simulink model "LATC_Test_Calc5"  (R2021b)
settings: Solver=FixedStepDiscrete  StartTime=4067.8601  StopTime=4107.8798  FixedStep=0.02  RelTol=1e-3
libraries: simulink x8
(part 1 of 2)
settings Model: DataDictionary=LATC.sldd  Creator=GW00216231  LastModifiedBy=GW00216231
settings SolverCC: AlgebraicLoopSolver=TrustRegion
settings OptimizationCC: DefaultParameterBehavior=Inlined  EnhancedBackFolding=on  PassReuseOutputArgsThreshold=0  OptimizeBlockOrder=speed  DifferentSizesBufferReuse=on  OptimizationCustomize=off
settings DebuggingCC: SignalResolutionControl=TryResolveAllWithWarning  ParameterTunabilityLossMsg=error  SFMachineParentedDataDiag=warning  UnderSpecifiedDimensionMsg=warning
settings SFSimCC: MATLABDynamicMemAlloc=off
settings RTWCC: Description=Vector CANape/vSignalyzer Target (Visual C/C++ Project Makefile)  SystemTargetFile=cnp.tlc  TemplateMakefile=cnp_msdll.tmf
settings CodeAppCC: ForceParamTrailComments=on  OperatorAnnotations=on
settings STFCustomTargetCC: TargetLangStandard=C99 (ISO)  MATLABClassNameForMDSCustomization=Simulink.SoftwareTarget.TargetSpecificTriggerConfigurationBase  SystemTargetFile=cnp.tlc

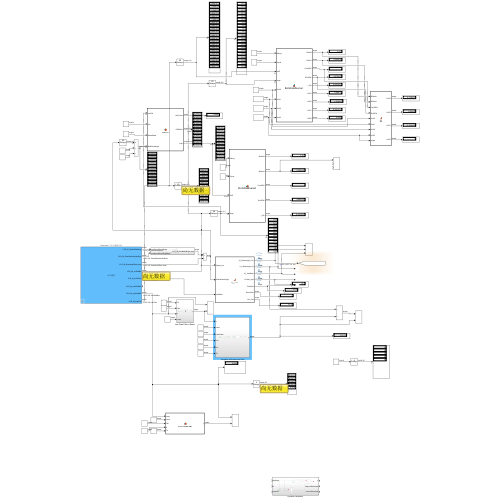
[thumbnail: Simulink's stored preview of the top-level diagram]
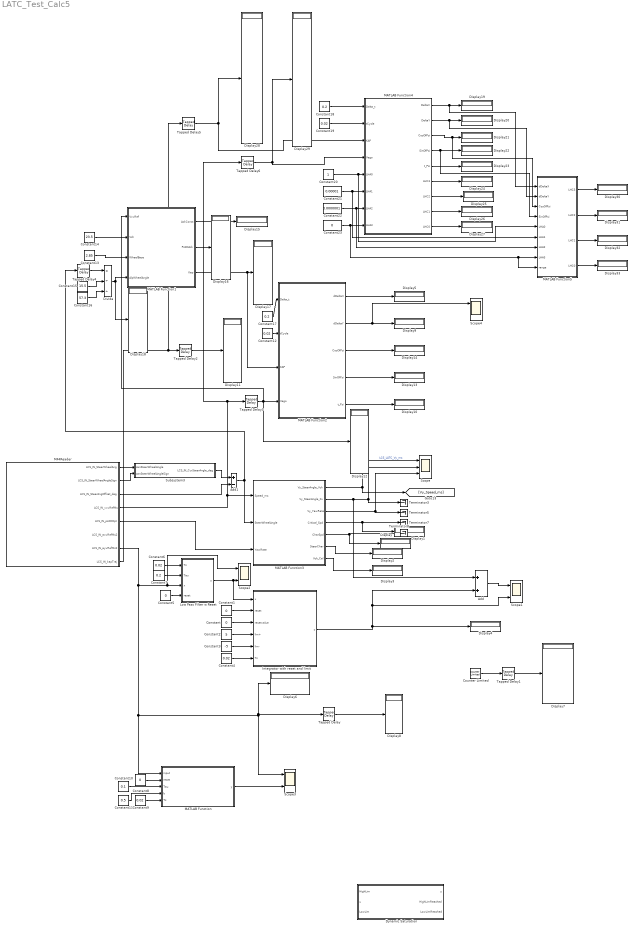
== system LATC_Test_Calc5 ==
  Add : Sum
  Add1 : Sum  Inputs=+-
  Constant{,1,5,8,23} (5 alike) : Constant  Value=0  OutDataTypeStr=single
  Constant10 : Constant  Value=0.1  OutDataTypeStr=single
  Constant11 : Constant  Value=0.5  OutDataTypeStr=single
  Constant{4,6,9,12,19} (5 alike) : Constant  Value=0.02  OutDataTypeStr=single
  Constant13 : Constant  Value=2.85  OutDataTypeStr=single
  Constant14 : Constant  Value=23.5  OutDataTypeStr=single
  Constant15 : Constant  Value=15.5  OutDataTypeStr=single
  Constant16 : Constant  Value=57.3  OutDataTypeStr=single
  Constant17 : Constant  Value=0.2  OutDataTypeStr=single
  Constant18 : Constant  Value=0.2  OutDataTypeStr=single
  Constant2 : Constant  Value=5  OutDataTypeStr=single
  Constant20 : Constant  OutDataTypeStr=single
  Constant21 : Constant  Value=0.00001  OutDataTypeStr=single
  Constant22 : Constant  Value=0.0000001  OutDataTypeStr=single
  Constant3 : Constant  Value=-5  OutDataTypeStr=single
  Constant7 : Constant  Value=0.2  OutDataTypeStr=single
  Counter Limited : simulink/Sources/Counter Limited  uplimit=65535  tsamp=-1
  Display{,1..33} (34 alike) : Display
  Divide : Product  Inputs=*//
  Dynamic Saturation : Subsystem
  Integrator with reset and limit : Subsystem
  Low Pass Filter w Reset : Subsystem
  MATLAB Function : MATLAB Function  TreatAsAtomicUnit=on
  MATLAB Function1 : MATLAB Function  TreatAsAtomicUnit=on
  MATLAB Function2 : MATLAB Function  TreatAsAtomicUnit=on
  MATLAB Function3 : MATLAB Function  TreatAsAtomicUnit=on
  MATLAB Function4 : MATLAB Function  TreatAsAtomicUnit=on
  MATLAB Function5 : MATLAB Function  TreatAsAtomicUnit=on
  MF4Reader : Subsystem  Description=Comment: 汇出有碰撞风险  mask(MF4Reader(Bata1.5)){pfileName=F:\04_APE_Temple_Files\ADAS_CAN+dll+SimulinkModel\TrajectoryPoints_Track_Test4\Data_Recorder\NOH_IDC_V71_0049_2022-05-27-19-39-31.mf4, LoadFilter={'Checksum','RollingCounter','AEB','HAVP_','^P_','BSW','Reserved','PACK','autosar','LM_','exec','fid_stat','g_swc','_PIL_','_TLJ_','_PP_','SPID','DMON','gen_init','JAPedObj','^MAC','CAN_DataFrame','DIAG','CAL'}, CaseSensitive=off, AutoDataTypeConvert=off, FunMod=读入模式, SearchSeed=LCS_*kap, BackGroundColorRead=lightBlue, BackGroundColorPort=white, StopTime=4107.8798, StartTime=4067.8601}
      mask prompts: pfileName "mf4文件:"; LoadFilter "加载过滤:"; CaseSensitive "搜索大小写敏感"; AutoDataTypeConvert "自动数据类型转换"; FunMod "模式选择"; SearchSeed "搜索："; StopTime "数据结束时间"; StartTime "数据开始时间"
      mask help: 该模块可将选择的mdf文件中包含的信号以列表形式读取出来，读入模式下，该模块将用户选择的信号读取成matlab时间序列，并导入simulink用于仿真。接口模式下，该模块将以用户选择的信号名添加CANape仿真用接口，用于dll生成（需要安装CANape simulink addon）。点击"帮助"了解更多。
      settings: AttributesFormatString=%<Description>
      mask Help:
      | Version：Bata1.5  Date: 20211012 Editor: Chengzhenning
      | 当前为测试版，可能存在不稳定或性能问题，建议/Bug反馈请联系Editor，谢谢。
      | 
      | 使用简述：
      | Step1:检查加载过滤。(若如特殊需求无需设置此项)
      | Step2:选取MF4文件
      | Setp3:点击Load/Refresh，加载mf4数据中的信号
      | Step4:选取信号（操作同bus selector，支持搜索）
      | Step5:选择模式及是否自动添加数据类型转换
      | Step6:点击Add添加接口
      | 
      | 数据导入：
      | 选择文件：支持mdf mf4文件，支持中文路径
      | 加载过滤：加载过滤是将符合过滤条件(标准matlab正则表达式)的所有信号跳过，过滤后在“全部信号”中无法找到，可配置多个过滤条件，多个条件以元胞数组的形式输入，例如{'表达式1'，'表达式2'} ，可根据情况自行修改。不建议删除默认的加载过滤条件。
      | 
      | 自定义设置项说明：
      | 读入模式：当配置为导入mdf数据后，该模块会将已选择的信号从mdf文件中读取出来，存入base workspace。并在模型中使用fromworkspace调用。
      | 接口模式：当配置为生成ape接口时，将按照已选择的信号名生成ape仿真用接口模块。
      | 自动数据类型转换：设置为自动数据类型转换之后将在内部自动添加data type conversion，请务必规定后端使用的数据类型，否者以读出或输入的数据类型直出。
      | 
      | 搜索：
      | 搜索：搜索支持常用通配符（同ape），当搜索条件为空或点击输入框的取消后将重置搜索结果，搜索条件请在弹出的输入框中输入；
      | 
      | 其他提醒：
      | 因版本限制，自定义设置部分请用右侧按钮进行设置，左侧仅作显示用；
      | 因版本限制，搜索条件请在弹出的输入框中输入；
      | 加载数据后，该模块会自动将仿真起止时间设置为所有有效数据的最大起止时间区间，仿真步长需要自行设置；
      | 
      | 故障解决：
      | 若发生接口混乱的情况，点击不常用设置->ClearPorts！删除所有模块后重新添加。
      | 若存在其他报错问题，尝试执行clear all（所有工作区将被清除，注意保存数据！！！）后重新load数据。
      | 若提醒找不到变，在没有clear all的前提下，重新Add即可。若执行了clear all，需要点击Load重新加载数据。
      | 
      | 兼容性：
      | 兼容20b和21a，但因2020b兼容性问题，部分参数只能使用对话框的形式输入而不能直接修改，Matlab 21a版本体验更佳。若需要21a版，请联系Editor。
      | 
      | 警告：
      | 删除默认的加载过滤条件可能会导致错误，不建议删除默认的加载过滤条件！
      | 每个模型中只能同时使用一个MF4Reader !
      | 尽量不要手动清空工作区，clear之后需求重新add，clear all之后需要重新load并add
      | 
      | 更新记录：
      | 1 Bata1.0  Date 20210927 Editor Chengzhenning
      |    初版发布
      | 2 Bata1.1  Date 20210929 Editor Chengzhenning
      |    优化个别无法读取的信号的检测过滤,提高对数据的兼容性，bug反馈人：温俊亮
      | 3 Bata1.2  Date 20210930 Editor Chengzhenning
      |    修复重调整接口会导致外部连线混乱的问题，不再使用弹窗提醒找不到的信号，bug反馈人：王亚伟
      | 4.Bata1.3  Date 20210930 Editor Chengzhenning
      |    自动添加信号名，提升加载数据速度
      | 5.Bata1.4  Date 20211009 Editor Chengzhenning
      |    增加内部的自动信号类型转换，可配置。支持设置搜索是否大小写敏感。更改设置工作模式的位置，不必每次都设置。
      | 6.Bata1.5  Date 20211012 Editor Chengzhenning
      |    适配2021b，不再兼容2020b以下。其他操作逻辑优化，更易使用。
      | 
      | 感谢所有提供bug反馈和功能建议的用户！
      mask TypeOptions FunMod: 读入模式 | 接口模式
      mask DialogControl ParameterGroupVar Prompt: 数据源选择
      mask DialogControl Control2 Prompt: 选择文件
      mask DialogControl Control2 Callback:
      | global fileobj;
      | 
      | [Name,directory] = uigetfile('*.mf4;*.mdf','Choose a mf4-file');
      | if isequal(Name,0) || isequal(directory,0)
      |     disp('User pressed cancel')
      |     return;
      | else
      |     fName=fullfile(directory,Name);
      |     if strcmp(fName,get_param(gcb,'pfileName'))&&~isempty(fileobj)
      |         return;
      |     end
      |     set_param(gcb,'pfileName',fName);
      |     disp(['User selected ',fName ])
      | end
      | 
      | 
      | commentStr=NaN;
      | StartTime=0;
      | StopTime=30;
      | if ~isempty(Simulink.Mask.get(gcb).Parameters(2).Value)
      |     LoadExclude=eval(Simulink.Mask.get(gcb).Parameters(2).Value);
      |     if ~iscell(LoadExclude)
      |         msgbox('加载过滤必须是元胞字符串数组或空值！');
      |         return;
      |     end
      | else
      |     LoadExclude={};
      | end
      | fName=Simulink.Mask.get(gcb).Parameters(1).Value;
      | if ~exist(fName)
      |     msgbox('文件不存在！');
      |     return;
      | end
      | t1=clock;
      | disp('-----------------------------');
      | disp(['打开文件:',fName,'中...']);
      | bar = waitbar(0,'正在读取数据...0%');
      | fileobj=mdf(fName);
      | disp(['打开完成，用时',num2str(etime(clock,t1)),'秒']);
      | %commentStr=native2unicode(unicode2native(fileobj.Comment,'windows-1252'));%20b以下版本用
      | commentStr=fileobj.Comment;
      | disp(['数据备注:',commentStr]);
      | t1=clock;
      | disp('读取信号中...');
      | ALLSigNames={};
      | ALLSigsGroup={};
      | ChannelNamesNum=length(fileobj.ChannelNames);
      | timeflag=true;
      | for i=2:ChannelNamesNum
      |     if ishandle(bar)
      |         str=['正在加载数据...',num2str(fix(100*i/ChannelNamesNum)),'%'];
      |         waitbar(i/ChannelNamesNum,bar,str,'Interpreter','none');
      |     end
      |     if fileobj.ChannelGroup(i).DataSize==0
      |         continue;
      |     end
      |     for m=1:length(fileobj.ChannelNames{i})
      |         ChannelName=fileobj.ChannelNames{i}{m};
      |         if (ChannelName=='t')
      |             continue;
      |         end
      |         if isempty(ChannelName)
      |             continue;
      |         end
      |         ExcludeFlag=false;
      |         for x=1:length(LoadExclude)
      |             if regexp(ChannelName,LoadExclude{x})
      |                 ExcludeFlag=true;
      |             end
      |         end
      |         if ExcludeFlag
      |             continue;
      |         end
      |         try
      |             temp=read(fileobj,i,ChannelName,'OutputFormat','Timeseries');
      |         catch
      |             disp([ChannelName,'不支持读入,已跳过！']);
      |         end
      |         if isempty(temp)
      |             continue;
      |         end
      |         timelength=temp.TimeInfo.end-temp.TimeInfo.start;
      |         if timelength<=0
      |             continue;
      |         end
      |         if timeflag
      |             StartTime=temp.TimeInfo.start;
      |             StopTime=temp.TimeInfo.end;
      |             timeflag=false;
      |         else
      |             if StartTime>temp.TimeInfo.start
      |                 StartTime=temp.TimeInfo.start;
      |             end
      |             if StopTime<temp.TimeInfo.end
      |                 StopTime=temp.TimeInfo.end;
      |             end
      |         end
      | 
      |         ALLSigNames=[ALLSigNames,ChannelName];
      |         ALLSigsGroup=[ALLSigsGroup,num2str(i)];
      |     end
      | end
      | 
      | %set_param(gcs,'StartTime',num2str(StartTime));
      | %set_param(gcs,'StopTime',num2str(StopTime));
      | set_param(gcb,'StartTime',num2str(StartTime));
      | set_param(gcb,'StopTime',num2str(StopTime));
      | waitbar(1,bar,['加载结束，信号数量：',num2str(length(ALLSigNames))],'Interpreter','none');
      | pause(2);
      | if ishandle(bar)
      |     close(bar);
      | end
      | if isempty(ALLSigNames)
      |     msgbox('读取数据失败！');
      |     disp('异常结束!');
      |     return;
      | else
      |     %commentStr=native2unicode(unicode2native(fileobj.Comment,'windows-1252'));
      |     disp(['读取完成,','信号数量：',num2str(length(ALLSigNames)),',用时',num2str(etime(clock,t1)),'秒']);
      |     disp(['数据起止时间为[',num2str(StartTime),' , ',num2str(StopTime),']']);
      |     disp('Finish!');
      | end
      | disp('-----------------------------');
      | set_param(gcb,'Description',['Comment: ',commentStr]);
      | 
      | 
      | maskObj = Simulink.Mask.get( gcb );
      | ControlALLSigsGroup= maskObj.getDialogControl('ALLSigsGroup');
      | ControlALLSigNames= maskObj.getDialogControl('ALLSigNames');
      | treeControlL = maskObj.getDialogControl('Control3');
      | treeControlR = maskObj.getDialogControl('Control6');
      | 
      | ControlALLSigsGroup.TreeItems=ALLSigsGroup;
      | ControlALLSigNames.TreeItems=ALLSigNames;
      | treeControlL.TreeItems=ALLSigNames;
      | 
      | selAllSig=treeControlR.TreeItems();
      | if isempty(selAllSig)
      |     return;
      | end
      | for i= 1:length(selAllSig)
      |     if max(strfind(selAllSig{i},'???'))>0
      |         if ismember(selAllSig{i}(4:end),ALLSigNames)
      |             selAllSig{i}=selAllSig{i}(4:end);
      |         end
      |     else
      |         if ~ismember(selAllSig{i},ALLSigNames)
      |             selAllSig{i}=['???',selAllSig{i}];
      |         end
      |     end
      | end
      | treeControlR.TreeItems=selAllSig;
      mask DialogControl Container11 Prompt: 自定义设置
      mask DialogControl SearchButton Prompt: Search
      mask DialogControl SearchButton Callback:
      | maskObj = Simulink.Mask.get( gcb );
      | treeControlL = maskObj.getDialogControl('Control3');
      | ControlALLSigNames= maskObj.getDialogControl('ALLSigNames');
      | ALLSigNames=ControlALLSigNames.TreeItems();
      | 
      | SearchSeed= get_param(gcb,'SearchSeed');
      | SearchSeed=strrep(SearchSeed,'[','');
      | SearchSeed=strrep(SearchSeed,']','');
      | SLsiglist={};
      | if isempty(SearchSeed)
      |     treeControlL.TreeItems=ALLSigNames;
      |     return;
      | end
      | CaseSensitive=get_param(gcb,'CaseSensitive');
      | if CaseSensitive=="off"
      |     for i=1:length(ALLSigNames)
      |         if regexpi(ALLSigNames{i},regexptranslate('wildcard',SearchSeed))
      |             %if regexp(ALLSigNames{i},SerchSeed)
      |             SLsiglist=[SLsiglist,ALLSigNames{i}];
      |         end
      |     end
      | else
      |     for i=1:length(ALLSigNames)
      |         if regexp(ALLSigNames{i},regexptranslate('wildcard',SearchSeed))
      |         %   if regexp(ALLSigNames{i},SerchSeed)
      |             SLsiglist=[SLsiglist,ALLSigNames{i}];
      |         end
      |     end
      | end
      | treeControlL.TreeItems=SLsiglist;
      mask DialogControl Control3 Prompt: 所有信号
      mask DialogControl Control9 Prompt: Load
      mask DialogControl Control9 Callback:
      | global fileobj;
      | 
      | commentStr=NaN;
      | StartTime=0;
      | StopTime=30;
      | if ~isempty(Simulink.Mask.get(gcb).Parameters(2).Value)
      |     LoadExclude=eval(Simulink.Mask.get(gcb).Parameters(2).Value);
      |     if ~iscell(LoadExclude)
      |         msgbox('加载过滤必须是元胞字符串数组或空值！');
      |         return;
      |     end
      | else
      |     LoadExclude={};
      | end
      | fName=Simulink.Mask.get(gcb).Parameters(1).Value;
      | if ~exist(fName)
      |     msgbox('文件不存在！');
      |     return;
      | end
      | t1=clock;
      | disp('-----------------------------');
      | disp(['打开文件:',fName,'中...']);
      | bar = waitbar(0,'正在读取数据...0%');
      | fileobj=mdf(fName);
      | disp(['打开完成，用时',num2str(etime(clock,t1)),'秒']);
      | %commentStr=native2unicode(unicode2native(fileobj.Comment,'windows-1252'));%20b以下版本用
      | commentStr=fileobj.Comment;
      | disp(['数据备注:',commentStr]);
      | t1=clock;
      | disp('读取信号中...');
      | ALLSigNames={};
      | ALLSigsGroup={};
      | ChannelNamesNum=length(fileobj.ChannelNames);
      | timeflag=true;
      | for i=2:ChannelNamesNum
      |     if ishandle(bar)
      |         str=['正在加载数据...',num2str(fix(100*i/ChannelNamesNum)),'%'];
      |         waitbar(i/ChannelNamesNum,bar,str,'Interpreter','none');
      |     end
      |     if fileobj.ChannelGroup(i).DataSize==0
      |         continue;
      |     end
      |     for m=1:length(fileobj.ChannelNames{i})
      |         ChannelName=fileobj.ChannelNames{i}{m};
      |         if (ChannelName=='t')
      |             continue;
      |         end
      |         if isempty(ChannelName)
      |             continue;
      |         end
      |         ExcludeFlag=false;
      |         for x=1:length(LoadExclude)
      |             if regexp(ChannelName,LoadExclude{x})
      |                 ExcludeFlag=true;
      |             end
      |         end
      |         if ExcludeFlag
      |             continue;
      |         end
      |         try
      |             temp=read(fileobj,i,ChannelName,'OutputFormat','Timeseries');
      |         catch
      |             disp([ChannelName,'不支持读入,已跳过！']);
      |         end
      |         if isempty(temp)
      |             continue;
      |         end
      |         timelength=temp.TimeInfo.end-temp.TimeInfo.start;
      |         if timelength<=0
      |             continue;
      |         end
      |         if timeflag
      |             StartTime=temp.TimeInfo.start;
      |             StopTime=temp.TimeInfo.end;
      |             timeflag=false;
      |         else
      |             if StartTime>temp.TimeInfo.start
      |                 StartTime=temp.TimeInfo.start;
      |             end
      |             if StopTime<temp.TimeInfo.end
      |                 StopTime=temp.TimeInfo.end;
      |             end
      |         end
      | 
      |         ALLSigNames=[ALLSigNames,ChannelName];
      |         ALLSigsGroup=[ALLSigsGroup,num2str(i)];
      |     end
      | end
      | 
      | %set_param(gcs,'StartTime',num2str(StartTime));
      | %set_param(gcs,'StopTime',num2str(StopTime));
      | set_param(gcb,'StartTime',num2str(StartTime));
      | set_param(gcb,'StopTime',num2str(StopTime));
      | waitbar(1,bar,['加载结束，信号数量：',num2str(length(ALLSigNames))],'Interpreter','none');
      | pause(2);
      | if ishandle(bar)
      |     close(bar);
      | end
      | if isempty(ALLSigNames)
      |     msgbox('读取数据失败！');
      |     disp('异常结束!');
      |     return;
      | else
      |     %commentStr=native2unicode(unicode2native(fileobj.Comment,'windows-1252'));
      |     disp(['读取完成,','信号数量：',num2str(length(ALLSigNames)),',用时',num2str(etime(clock,t1)),'秒']);
      |     disp(['数据起止时间为[',num2str(StartTime),' , ',num2str(StopTime),']']);
      |     disp('Finish!');
      | end
      | disp('-----------------------------');
      | set_param(gcb,'Description',['Comment: ',commentStr]);
      | 
      | 
      | maskObj = Simulink.Mask.get( gcb );
      | ControlALLSigsGroup= maskObj.getDialogControl('ALLSigsGroup');
      | ControlALLSigNames= maskObj.getDialogControl('ALLSigNames');
      | treeControlL = maskObj.getDialogControl('Control3');
      | treeControlR = maskObj.getDialogControl('Control6');
      | 
      | ControlALLSigsGroup.TreeItems=ALLSigsGroup;
      | ControlALLSigNames.TreeItems=ALLSigNames;
      | treeControlL.TreeItems=ALLSigNames;
      | 
      | selAllSig=treeControlR.TreeItems();
      | if isempty(selAllSig)
      |     return;
      | end
      | for i= 1:length(selAllSig)
      |     if max(strfind(selAllSig{i},'???'))>0
      |         if ismember(selAllSig{i}(4:end),ALLSigNames)
      |             selAllSig{i}=selAllSig{i}(4:end);
      |         end
      |     else
      |         if ~ismember(selAllSig{i},ALLSigNames)
      |             selAllSig{i}=['???',selAllSig{i}];
      |         end
      |     end
      | end
      | treeControlR.TreeItems=selAllSig;
      mask DialogControl Control7 Prompt: Select >>
      mask DialogControl Control7 Callback:
      | maskObj = Simulink.Mask.get( gcb );
      | treeControlL = maskObj.getDialogControl('Control3');
      | treeControlR = maskObj.getDialogControl('Control6');
      | 
      | seld=treeControlL.getSelectedItems();
      | if isempty(seld)
      |     return;
      | end
      | if ismember(seld,treeControlR.TreeItems)
      |     msgbox('信号重复')
      | end
      | treeControlR.TreeItems=unique([treeControlR.TreeItems,seld'],'stable');
      | treeControlR.setSelectedItems(seld);
      mask DialogControl Control6 Prompt: 已选信号
      mask DialogControl up Prompt: Up
      mask DialogControl up Callback:
      | maskObj = Simulink.Mask.get(gcb);
      | treeControlR = maskObj.getDialogControl('Control6');
      | RSig=treeControlR.TreeItems();
      | SelectSig=treeControlR.getSelectedItems();
      | 
      | if isempty(SelectSig)
      |     return;
      | end
      | 
      | [~,selIndex]=ismember(SelectSig,RSig);
      | 
      | if min(selIndex)>2
      |     AllSigPart3=RSig(1:min(selIndex)-2);
      | else
      |     AllSigPart3={};
      | end
      | RSig(selIndex)=[];
      | [~,Part1Index]=ismember(AllSigPart3,RSig);
      | RSig(Part1Index)=[];
      | 
      | treeControlR.TreeItems=[AllSigPart3,SelectSig',RSig];
      | treeControlR.setSelectedItems(SelectSig);
      mask DialogControl down Prompt: Down
      mask DialogControl down Callback:
      | maskObj = Simulink.Mask.get(gcb);
      | treeControlR = maskObj.getDialogControl('Control6');
      | RSig=treeControlR.TreeItems();
      | SelectSig=treeControlR.getSelectedItems();
      | 
      | if isempty(SelectSig)
      |     return;
      | end
      | 
      | [~,selIndex]=ismember(SelectSig,RSig);
      | 
      | if max(selIndex)+2<=length(RSig)
      |     AllSigPart3=RSig(max(selIndex)+2:end);
      | else
      |     AllSigPart3={};
      | end
      | RSig(selIndex)=[];
      | [~,Part3Index]=ismember(AllSigPart3,RSig);
      | RSig(Part3Index)=[];
      | 
      | treeControlR.TreeItems=[RSig,SelectSig',AllSigPart3];
      | treeControlR.setSelectedItems(SelectSig);
      mask DialogControl Control11 Prompt: Remove
      mask DialogControl Control11 Callback:
      | maskObj = Simulink.Mask.get(gcb);
      | treeControlR = maskObj.getDialogControl('Control6');
      | AllSig=treeControlR.TreeItems();
      | SelectSig=treeControlR.getSelectedItems();
      | if ~isempty(SelectSig)
      |     [~,DelIndex]=ismember(SelectSig,AllSig);
      |     AllSig(DelIndex)=[];
      | end
      | treeControlR.TreeItems=AllSig;
      mask DialogControl Control8 Prompt: Add
      mask DialogControl Control8 Callback:
      | global fileobj
      | if isempty(fileobj)
      |     msgbox('数据丢失，请重新load！');
      |     return;
      | end
      | FunMod=get_param(gcb,'FunMod');
      | %检查是否存在未识别到的信号
      | maskObj = Simulink.Mask.get( gcb );
      | treeControlL = maskObj.getDialogControl('Control3');
      | treeControlR = maskObj.getDialogControl('Control6');
      | ControlALLSigsGroup= maskObj.getDialogControl('ALLSigsGroup');
      | ControlALLSigNames= maskObj.getDialogControl('ALLSigNames');
      | ControlOldSigName= maskObj.getDialogControl('OldSigName');
      | 
      | DataSelect=treeControlR.TreeItems();
      | ALLSigsGroup=ControlALLSigsGroup.TreeItems();
      | ALLSigNames=ControlALLSigNames.TreeItems();
      | OldSigName=ControlOldSigName.TreeItems();
      | 
      | if isempty(DataSelect)
      |     msgbox('未选择信号！');
      |     return;
      | end
      | if isempty(DataSelect)
      |     return;
      | end
      | if ~iscell(ALLSigNames)
      |     ALLSigNames={};
      | end
      | for i= 1:length(DataSelect)
      |     if max(strfind(DataSelect{i},'???'))>0
      |         if ismember(DataSelect{i}(4:end),ALLSigNames)
      |             DataSelect{i}=DataSelect{i}(4:end);
      |         end
      |     else
      |         if ~ismember(DataSelect{i},ALLSigNames)
      |             DataSelect{i}=['???',DataSelect{i}];
      |         end
      |     end
      | end
      | treeControlR.TreeItems=DataSelect;
      | signotfind=false;
      | for i= 1:length(DataSelect)
      |     if max(strfind(DataSelect{i},'???'))>0
      |         signotfind=true;
      |     end
      | end
      | if signotfind
      |     signotfindresp=questdlg('存在已选的信号无法找到！请刷新数据或检查数据中是否存在这些信号','错误提醒','跳过无法找到的信号','停止添加接口','停止添加接口');
      |     if isempty(signotfindresp) || signotfindresp == "停止添加接口"
      |         return;
      |     end
      | end
      | 
      | oldPos=get_param(gcb,'Position');%记忆位置，防止游走
      | %定义模块路径方便使用
      | FunctionBlockPath = 'simulink/User-Defined Functions/Interpreted MATLAB Function';
      | OutPortBlockPath ='simulink/Commonly Used Blocks/Out1';
      | SaturationPath ='simulink/Discontinuities/Saturation';
      | ConstantPath = 'simulink/Sources/Constant';
      | DIPath = 'simulink/Discrete/Discrete-Time Integrator';
      | FromWorkSpacePath = 'simulink/Sources/From Workspace';
      | CANapeInputPath='canapelib/CANape I//O/Input';
      | DataTypeConversionPath='simulink/Signal Attributes/Data Type Conversion';
      | 
      | %添加模块前先删除所有模块和连线
      | set_param(gcb,'BackGroundColor','white');
      | SourceList=find_system(gcb,'LookUnderMasks','on','SearchDepth',1,'BlockType','FromWorkspace');
      | if ~isempty(SourceList)
      |     for i=1:length(SourceList)
      |         delete_block(SourceList{i});
      |     end
      | end
      | LinesList=find_system(gcb,'LookUnderMasks','on','FindAll','on','type','line');
      | if ~isempty(LinesList)
      |     for i=1:length(LinesList)
      |         if ishandle(LinesList(i))
      |             delete_line(LinesList(i));
      |         end
      |     end
      | end
      | 
      | SysList=find_system(gcb,'LookUnderMasks','on','SearchDepth',1,'BlockType','SubSystem');
      | if length(SysList)>1
      |     for i=2:length(SysList)
      |         delete_block(SysList{i});
      |     end
      | end
      | DataTypeConversionsList=find_system(gcb,'LookUnderMasks','on','SearchDepth',1,'BlockType','DataTypeConversion');
      | if ~isempty(DataTypeConversionsList)
      |     for i=1:length(DataTypeConversionsList)
      |         delete_block(DataTypeConversionsList{i});
      |     end
      | end
      | %添加信号源
      | SourceBlockSum=0;
      | added_block={};
      | if ~isempty(OldSigName)
      |     for i=1:length(OldSigName);
      |         evalin('base',['clear ',OldSigName{i}]);
      |     end
      | end
      | AutoDataTypeConvert=get_param(gcb,'AutoDataTypeConvert');
      | 
      | if FunMod=="读入模式" %fromworkspace
      |     for j=1:length(DataSelect)
      |         SigName=DataSelect{j};
      |         temp=strrep(SigName,'.','_');
      |         temp=strrep(temp,'[','_');
      |         temp=strrep(temp,']','_');
      |         if length(temp)>60
      |             temp=temp(length(temp)-59:end);
      |         end
      |         SigAliasName=['s_',temp];
      |         [SigExist,Sigindex]= ismember(SigName,ALLSigNames);
      |         if SigExist
      |             sigGroupIndex=str2double(ALLSigsGroup{Sigindex});
      |         else
      |             disp(['未找到信号: ',SigName,' ，已跳过！']);
      |             continue;
      |         end
      |         %添加模块
      |         Swidth=100;
      |         Shigh=30;
      |         Owidth=30;
      |         Ohigh=14;
      |         Sdy=30;
      |         SOdx=800;
      |         SDdx=250;
      |         temp=read(fileobj,sigGroupIndex,SigName,'OutputFormat','Timeseries');
      |         assignin('base',SigAliasName,temp);
      |         Source=add_block(FromWorkSpacePath,[gcb,'/' ,'sourceValue_',SigName],'Interpolate','off','VariableName',SigAliasName,'OutputAfterFinalValue','Setting to zero', ...
      |             'Position',[0,(Shigh)*SourceBlockSum+SourceBlockSum*Sdy, Swidth ,(Shigh)*(SourceBlockSum+1)+SourceBlockSum*Sdy]);
      |         if AutoDataTypeConvert=="on"
      |             DataTypeConversion=add_block(DataTypeConversionPath,[gcb,'/' ,'Convert_',SigName], ...
      |                 'Position',[SDdx,(Shigh)*SourceBlockSum+SourceBlockSum*Sdy, SDdx+Swidth ,(Shigh)*(SourceBlockSum+1)+SourceBlockSum*Sdy]);
      |         end
      |         Out=find_system(gcb,'LookUnderMasks','on','SearchDepth',1,'BlockType','Outport','PortName',SigName);
      |         if isempty(Out)
      |             Out=add_block(OutPortBlockPath,[gcb,'/' ,SigName],...
      |                 'Position',[SOdx,0.5*(Shigh-Ohigh)+(Ohigh)*SourceBlockSum+SourceBlockSum*(Sdy+Shigh-Ohigh),SOdx+Owidth ,0.5*(Shigh-Ohigh)+(Ohigh)*(SourceBlockSum+1)+SourceBlockSum*(Sdy+Shigh-Ohigh)]);
      |         else
      |             Out=Out{1};
      |             set_param(Out,'Port',num2str(SourceBlockSum+1),'Position',[SOdx,0.5*(Shigh-Ohigh)+(Ohigh)*SourceBlockSum+SourceBlockSum*(Sdy+Shigh-Ohigh),SOdx+Owidth ,0.5*(Shigh-Ohigh)+(Ohigh)*(SourceBlockSum+1)+SourceBlockSum*(Sdy+Shigh-Ohigh)]);
      |         end
      |         if AutoDataTypeConvert=="on"
      |             add_line(gcb,get_param(Source,'PortHandles').Outport,get_param(DataTypeConversion,'PortHandles').Inport)
      |             line=add_line(gcb,get_param(DataTypeConversion,'PortHandles').Outport,get_param(Out,'PortHandles').Inport);
      |         else
      |             line=add_line(gcb,get_param(Source,'PortHandles').Outport,get_param(Out,'PortHandles').Inport);
      |         end
      |         set_param(line,'Name',SigName);
      |         SourceBlockSum=SourceBlockSum+1;
      |         set_param(get_param(gcb,'PortHandles').Outport(SourceBlockSum),'ShowPropagatedSignals','on');
      |         OldSigName{j}=SigAliasName;
      |     end
      |     set_param(gcb,'BackGroundColor',get_param(gcb,'BackGroundColorRead'));
      |     set_param(gcs,'StartTime',get_param(gcb,'StartTime'));
      |     set_param(gcs,'StopTime',get_param(gcb,'StopTime'));
      |     disp('读入数据完成，已经自动设置模型仿真时间为数据起止时间');
      | elseif FunMod=="接口模式"
      |     for j=1:length(DataSelect)
      |         SigName=DataSelect{j};
      |         temp=strrep(SigName,'.','_');
      |         if length(temp)>60
      |             temp=temp(length(temp)-59:end);
      |         end
      |         SigAliasName=['s_',temp];
      |         [SigExist,Sigindex]= ismember(SigName,ALLSigNames);
      |         if SigExist
      |             sigGroupIndex=ALLSigsGroup{Sigindex};
      |         else
      |             disp(['未找到信号: ',SigName,' ，已跳过！']);
      |             continue
      |         end
      |         %添加模块
      |         Swidth=100;
      |         Shigh=30;
      |         Owidth=30;
      |         Ohigh=14;
      |         Sdy=30;
      |         SOdx=800;
      |         SDdx=250;
      |         try
      |         Source=add_block('canapelib/CANape I//O/Input',[gcb,'/' ,'sourceValue_',SigName],...
      |             'envName',SigName,'Position',[0,(Shigh)*SourceBlockSum+SourceBlockSum*Sdy, Swidth ,(Shigh)*(SourceBlockSum+1)+SourceBlockSum*Sdy]);
      |         catch
      |             msgbox('可能未安装CANape Simulink Add-on！无法添加接口，已终止！')
      |             return;
      |         end
      |         if AutoDataTypeConvert=="on"
      |             DataTypeConversion=add_block(DataTypeConversionPath,[gcb,'/' ,'Convert_',SigName], ...
      |                 'Position',[SDdx,(Shigh)*SourceBlockSum+SourceBlockSum*Sdy-10, SDdx+Swidth ,(Shigh)*(SourceBlockSum+1)+SourceBlockSum*Sdy-10]);
      |         end
      |         Out=find_system(gcb,'LookUnderMasks','on','SearchDepth',1,'BlockType','Outport','PortName',SigName);
      |         if isempty(Out)
      |             Out=add_block(OutPortBlockPath,[gcb,'/' ,SigName],...
      |                 'Position',[SOdx,0.5*(Shigh-Ohigh)+(Ohigh)*SourceBlockSum+SourceBlockSum*(Sdy+Shigh-Ohigh)-10,SOdx+Owidth ,0.5*(Shigh-Ohigh)+(Ohigh)*(SourceBlockSum+1)+SourceBlockSum*(Sdy+Shigh-Ohigh)-10]);
      |         else
      |             Out=Out{1};
      |             set_param(Out,'Port',num2str(SourceBlockSum+1),'Position',[SOdx,0.5*(Shigh-Ohigh)+(Ohigh)*SourceBlockSum+SourceBlockSum*(Sdy+Shigh-Ohigh)-10,SOdx+Owidth ,0.5*(Shigh-Ohigh)+(Ohigh)*(SourceBlockSum+1)+SourceBlockSum*(Sdy+Shigh-Ohigh)-10]);
      |         end
      |         if AutoDataTypeConvert=="on"
      |             add_line(gcb,get_param(Source,'PortHandles').Outport(1),get_param(DataTypeConversion,'PortHandles').Inport)
      |             line=add_line(gcb,get_param(DataTypeConversion,'PortHandles').Outport,get_param(Out,'PortHandles').Inport);
      |         else
      |             line=add_line(gcb,get_param(Source,'PortHandles').Outport(1),get_param(Out,'PortHandles').Inport);
      |         end
      |         set_param(line,'Name',SigName);
      |         SourceBlockSum=SourceBlockSum+1;
      |         set_param(get_param(gcb,'PortHandles').Outport(SourceBlockSum),'ShowPropagatedSignals','on');
      |         OldSigName{j}=SigAliasName;
      |     end
      |     set_param(gcb,'BackGroundColor',get_param(gcb,'BackGroundColorPort'));
      |     set_param(gcs,'StartTime','0');
      |     disp('添加CANape接口完成，已经自动设置模型仿真开始时间为0');
      | end
      | ControlOldSigName.TreeItems=OldSigName;
      | % 删除多余output
      | OutList=find_system(gcb,'LookUnderMasks','on','SearchDepth',1,'BlockType','Outport');
      | if ~isempty(OutList)
      |     for i=1:length(OutList)
      |         if str2double(get_param(OutList{i},'Port'))>SourceBlockSum
      |             delete_block(OutList{i});
      |         end
      |     end
      | end
      | 
      | if (oldPos(4)-oldPos(2))/SourceBlockSum<20
      |     oldPos(4)=oldPos(2)+(SourceBlockSum+1)*20;
      | end
      | set_param(gcb,'Position',oldPos);
      mask DialogControl ccc Prompt: 其他不常用设置
      mask DialogControl Control17 Prompt: 记忆当前模式模块颜色
      mask DialogControl Control17 Callback:
      | FunMod=get_param(gcb,'FunMod');
      | if FunMod=="读入模式"
      |     set_param(gcb,'BackGroundColorRead',get_param(gcb,'BackGroundColor'));
      | end
      | if FunMod=="接口模式"
      |     set_param(gcb,'BackGroundColorPort',get_param(gcb,'BackGroundColor'));
      | end
      mask DialogControl Control25 Prompt: ClearPorts!
      mask DialogControl Control25 Callback:
      | SourceList=find_system(gcb,'LookUnderMasks','on','SearchDepth',1,'BlockType','FromWorkspace');
      | if ~isempty(SourceList)
      |     for i=1:length(SourceList)
      |         delete_block(SourceList{i});
      |     end
      | end
      | LinesList=find_system(gcb,'LookUnderMasks','on','FindAll','on','type','line');
      | if ~isempty(LinesList)
      |     for i=1:length(LinesList)
      |         if ishandle(LinesList(i))
      |             delete_line(LinesList(i));
      |         end
      |     end
      | end
      | 
      | SysList=find_system(gcb,'LookUnderMasks','on','SearchDepth',1,'BlockType','SubSystem');
      | if length(SysList)>1
      |     for i=2:length(SysList)
      |         delete_block(SysList{i});
      |     end
      | end
      | DataTypeConversionsList=find_system(gcb,'LookUnderMasks','on','SearchDepth',1,'BlockType','DataTypeConversion');
      | if ~isempty(DataTypeConversionsList)
      |     for i=1:length(DataTypeConversionsList)
      |         delete_block(DataTypeConversionsList{i});
      |     end
      | end
      | OutList=find_system(gcb,'LookUnderMasks','on','SearchDepth',1,'BlockType','Outport');
      | if ~isempty(OutList)
      |     for i=1:length(OutList)
      |         delete_block(OutList{i});
      |     end
      | end
      mask DialogControl Container13 Prompt: Debug
      mask DialogControl OldSigName Prompt: OldSigName
      mask DialogControl ALLSigNames Prompt: ALLSigNames
      mask DialogControl ALLSigsGroup Prompt: ALLSigsGroup
      mask Display:
      | FunMod=get_param(gcb,'FunMod');
      | SourceList=find_system(gcb,'LookUnderMasks','on','SearchDepth',1,'BlockType','FromWorkspace');
      | SysList=find_system(gcb,'LookUnderMasks','on','SearchDepth',1,'BlockType','SubSystem');
      | if ~isempty(SourceList)
      | disp('读入模式');
      | elseif length(SysList)>1
      |     disp('接口模式');
      | else
      |     disp('未添加接口');
      | end
  Scope : Scope  NumInputPorts=3
  Scope1 : Scope  NumInputPorts=2
  Scope2 : Scope  NumInputPorts=2
  Scope3 : Scope  NumInputPorts=2
  Scope4 : Scope  NumInputPorts=3
  Subsystem3 : Subsystem
  Tapped Delay : simulink/Discrete/Tapped Delay  vinit=0.0  samptime=-1  NumDelays=4  DelayOrder=Oldest  includeCurrent=on
  Tapped Delay1 : simulink/Discrete/Tapped Delay  vinit=0.0  samptime=-1  NumDelays=4  DelayOrder=Newest  includeCurrent=on
  Tapped Delay{2..6} (5 alike) : simulink/Discrete/Tapped Delay  vinit=0.0  samptime=-1  NumDelays=20  DelayOrder=Oldest  includeCurrent=on
  Terminator{3,5,7..8} (4 alike) : Terminator
  wires:
  MATLAB Function3/5(CharSpd) -> Display/1, Terminator8/1
  MATLAB Function3/3(Vy_YawRate) -> Terminator5/1, Scope/3
  MATLAB Function3/2(Vy_SteerAngle_Kv) -> Add/1, Terminator3/1, Scope/2
  MATLAB Function3/1(Vy_SteerAngle_Vch) -> [Vy_Speed_ms], Scope/1  "LCS_LATC_Vy_ms"
  Add1/1 -> MATLAB Function3/2(SteerWheelAngle), Tapped Delay4/1
  MATLAB Function3/4(Critical_Spd) -> Display1/1, Terminator7/1
  MF4Reader/5(LCS_IN_psiDtOpt) -> MATLAB Function3/3(YawRate)
  MF4Reader/4(LCS_IN_vxvRefMs) -> MATLAB Function3/1(Speed_ms), Tapped Delay3/1, Tapped Delay6/1
  MF4Reader/1(LCS_IN_SteerWheelAng) -> Subsystem3/1(canSteerWheelAngle)
  MF4Reader/2(LCS_IN_SteerWheelAngleSign) -> Subsystem3/2(canSteerWheelAngleSign)
  Subsystem3/1(LCS_IN_CurSteerAngle_deg) -> Add1/1
  MF4Reader/3(LCS_IN_SteerAngOffset_deg) -> Add1/2
  MATLAB Function3/6(SteerChar) -> Display2/1
  MATLAB Function3/7(Vch_Cal) -> Display3/1
  Constant/1 -> Integrator with reset and limit/3(resetvalue)
  Constant1/1 -> Integrator with reset and limit/2(reset)
  Constant2/1 -> Integrator with reset and limit/4(lim+)
  Constant3/1 -> Integrator with reset and limit/5(lim-)
  Constant4/1 -> Integrator with reset and limit/6(Ts)
  Integrator with reset and limit/1(y) -> Add/2, Scope1/2, Display4/1
  Constant5/1 -> Low Pass Filter w Reset/4(reset)
  Low Pass Filter w Reset/1(y) -> Integrator with reset and limit/1(x), Scope2/2
  Constant6/1 -> Low Pass Filter w Reset/1(Ts)
  Constant7/1 -> Low Pass Filter w Reset/2(Tau)
  Add/1 -> Scope1/1
  Constant8/1 -> MATLAB Function/2(reset)
  Constant9/1 -> MATLAB Function/5(Ts)
  Constant10/1 -> MATLAB Function/3(Tau)
  Constant11/1 -> MATLAB Function/4(b)
  MATLAB Function/1(y) -> Scope3/2
  Tapped Delay/1 -> Display8/1
  MF4Reader/7(LCS_IN_ayvRefMs2) -> Display6/1, Tapped Delay/1, Scope3/1, MATLAB Function/1(input), Low Pass Filter w Reset/3(x), Scope2/1
  Counter Limited/1 -> Tapped Delay1/1
  Tapped Delay1/1 -> Display7/1
  Tapped Delay2/1 -> Display11/1
  Constant12/1 -> MATLAB Function2/2(tCycle)
  Tapped Delay3/1 -> MATLAB Function1/1(VxvRef), MATLAB Function2/4(Vego), Display12/1
  MATLAB Function2/1(dDeltaX) -> Display5/1
  MATLAB Function2/2(dDeltaY) -> Scope4/1, Display9/1
  MATLAB Function2/5(t_Psi) -> Display10/1
  MATLAB Function2/4(SinOfPsi) -> Display13/1
  MATLAB Function2/3(CosOfPsi) -> Display14/1
  Constant13/1 -> MATLAB Function1/3(WheelBase)
  Constant14/1 -> MATLAB Function1/2(Vch)
  Tapped Delay4/1 -> Divide/1
  Constant15/1 -> Divide/2
  Constant16/1 -> Divide/3
  MATLAB Function1/1(AckConst) -> Display15/1
  MATLAB Function1/2(PsiDtAck) -> Display16/1
  MATLAB Function1/3(Kap) -> MATLAB Function2/3(KAP), Display17/1
  Divide/1 -> Display18/1, MATLAB Function1/4(AlpWheelAngle)
  Constant17/1 -> MATLAB Function2/1(Delta_t)
  Constant18/1 -> MATLAB Function4/1(Delta_t)
  Constant19/1 -> MATLAB Function4/2(tCycle)
  Constant20/1 -> MATLAB Function5/5(LHA0), MATLAB Function4/5(LHA0)
  Constant21/1 -> MATLAB Function5/6(LHA1), MATLAB Function4/6(LHA1)
  Constant22/1 -> MATLAB Function5/7(LHA2), MATLAB Function4/7(LHA2)
  Constant23/1 -> MATLAB Function5/9(range), MATLAB Function5/8(LHA3), MATLAB Function4/8(LHA3)
  MATLAB Function4/1(DeltaX) -> MATLAB Function5/1(dDeltaX), Display19/1
  MATLAB Function4/2(DeltaY) -> MATLAB Function5/2(dDeltaY), Display20/1
  MATLAB Function4/3(CosOfPsi) -> MATLAB Function5/3(CosOfPsi), Display21/1
  MATLAB Function4/4(SinOfPsi) -> MATLAB Function5/4(SinOfPsi), Display22/1
  MATLAB Function4/5(t_Psi) -> Display23/1
  MATLAB Function4/6(LHC3) -> Display24/1
  MATLAB Function4/7(LHC2) -> Display25/1
  MATLAB Function4/8(LHC1) -> Display26/1
  MATLAB Function4/9(LHC0) -> Display27/1
  MF4Reader/8(LCS_IN_kapTraj) -> Tapped Delay2/1, Tapped Delay5/1
  Tapped Delay5/1 -> MATLAB Function4/3(KAP), Display28/1
  Tapped Delay6/1 -> MATLAB Function4/4(Vego), Display29/1
  MATLAB Function5/1(LHC3) -> Display30/1
  MATLAB Function5/2(LHC2) -> Display31/1
  MATLAB Function5/3(LHC1) -> Display32/1
  MATLAB Function5/4(LHC0) -> Display33/1

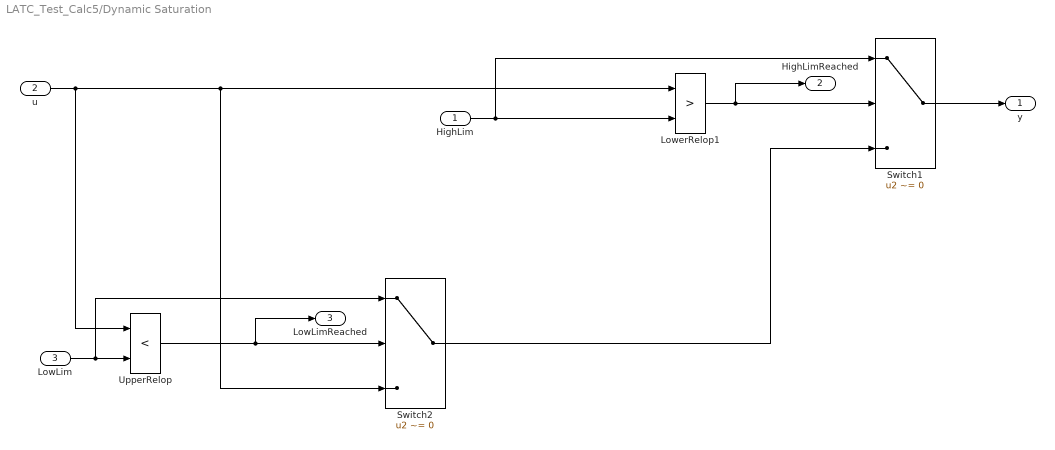
== system LATC_Test_Calc5/Dynamic Saturation ==
  HighLim : Inport
  u : Inport  Port=2
  LowLim : Inport  Port=3
  LowerRelop1 : RelationalOperator  DisableCoverage=on  Operator=>  OutDataTypeStr=boolean  RndMeth=Nearest
  Switch1 : Switch  Criteria=u2 ~= 0  InputSameDT=on
      settings: AttributesFormatString=InputSameDT = %<InputSameDT>
  Switch2 : Switch  Criteria=u2 ~= 0  InputSameDT=on
      settings: AttributesFormatString=InputSameDT = %<InputSameDT>
  UpperRelop : RelationalOperator  DisableCoverage=on  Operator=<  OutDataTypeStr=boolean  RndMeth=Nearest
  y : Outport
  HighLimReached : Outport  Port=2
  LowLimReached : Outport  Port=3
  wires:
  u/1 -> Switch2/3, LowerRelop1/1, UpperRelop/1
  HighLim/1 -> Switch1/1, LowerRelop1/2
  Switch1/1 -> y/1
  LowerRelop1/1 -> HighLimReached/1, Switch1/2
  UpperRelop/1 -> LowLimReached/1, Switch2/2
  Switch2/1 -> Switch1/3
  LowLim/1 -> Switch2/1, UpperRelop/2

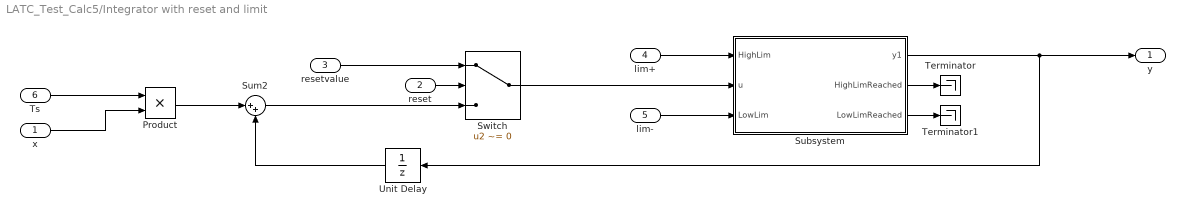
== system LATC_Test_Calc5/Integrator with reset and limit ==
  x : Inport
  reset : Inport  Port=2
  resetvalue : Inport  Port=3
  lim+ : Inport  Port=4
  lim- : Inport  Port=5
  Ts : Inport  Port=6
  Product : Product  RndMeth=Zero
  Subsystem : Subsystem
  Sum2 : Sum  Inputs=|++
  Switch : Switch  Criteria=u2 ~= 0
  Terminator : Terminator
  Terminator1 : Terminator
  Unit Delay : UnitDelay  SampleTime=-1  HasFrameUpgradeWarning=on
  y : Outport
  wires:
  Unit Delay/1 -> Sum2/2
  lim-/1 -> Subsystem/3(LowLim)
  Subsystem/1(y1) -> y/1, Unit Delay/1
  resetvalue/1 -> Switch/1
  Subsystem/2(HighLimReached) -> Terminator/1
  Ts/1 -> Product/1
  Sum2/1 -> Switch/3
  reset/1 -> Switch/2
  Product/1 -> Sum2/1
  x/1 -> Product/2
  Switch/1 -> Subsystem/2(u)
  lim+/1 -> Subsystem/1(HighLim)
  Subsystem/3(LowLimReached) -> Terminator1/1

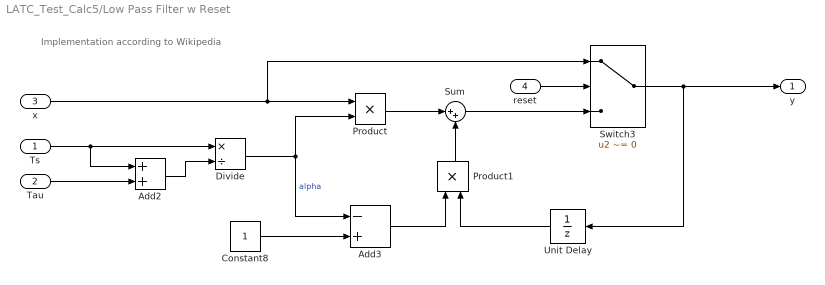
== system LATC_Test_Calc5/Low Pass Filter w Reset ==
  note: Implementation according to Wikipedia
  Ts : Inport
  Tau : Inport  Port=2
  x : Inport  Port=3
  reset : Inport  Port=4
  Add2 : Sum
  Add3 : Sum  Inputs=-+
  Constant8 : Constant  OutDataTypeStr=single
  Divide : Product  Inputs=*/
  Product : Product  RndMeth=Zero
  Product1 : Product  RndMeth=Zero
  Sum : Sum  Inputs=|++
  Switch3 : Switch  Criteria=u2 ~= 0
  Unit Delay : UnitDelay  SampleTime=-1  HasFrameUpgradeWarning=on
  y : Outport  PortDimensions=1
  wires:
  Add3/1 -> Product1/1
  Product1/1 -> Sum/2
  x/1 -> Switch3/1, Product/1
  Product/1 -> Sum/1
  Ts/1 -> Divide/1, Add2/1
  Unit Delay/1 -> Product1/2
  Add2/1 -> Divide/2
  Divide/1 -> Product/2, Add3/1  "alpha"
  reset/1 -> Switch3/2
  Sum/1 -> Switch3/3
  Constant8/1 -> Add3/2
  Tau/1 -> Add2/2
  Switch3/1 -> y/1, Unit Delay/1

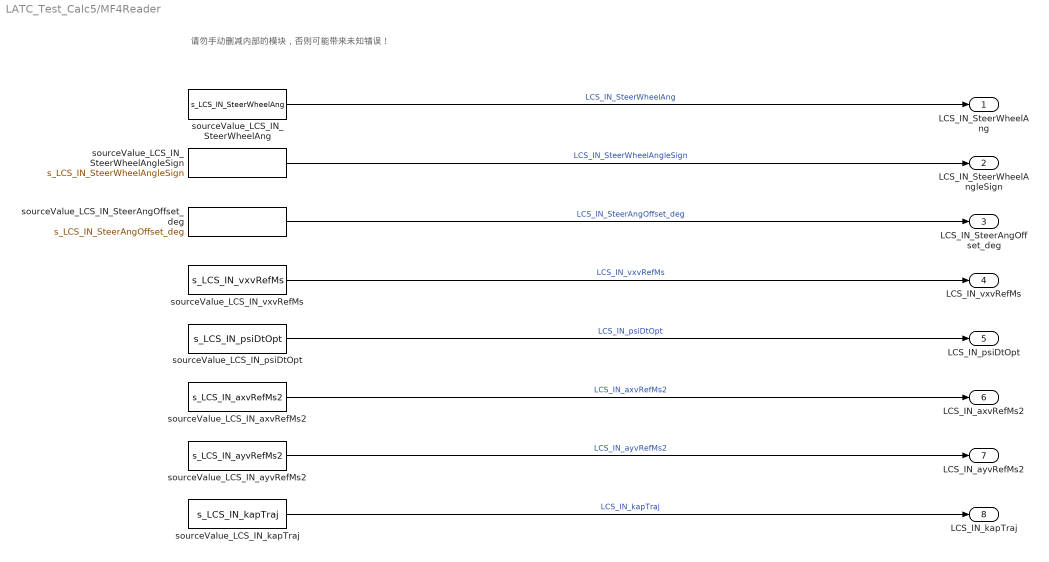
== system LATC_Test_Calc5/MF4Reader ==
  note: 请勿手动删减内部的模块，否则可能带来未知错误！
  sourceValue_LCS_IN_SteerAngOffset_deg : FromWorkspace  VariableName=s_LCS_IN_SteerAngOffset_deg  Interpolate=off  OutputAfterFinalValue=Setting to zero
  sourceValue_LCS_IN_SteerWheelAng : FromWorkspace  VariableName=s_LCS_IN_SteerWheelAng  Interpolate=off  OutputAfterFinalValue=Setting to zero
  sourceValue_LCS_IN_SteerWheelAngleSign : FromWorkspace  VariableName=s_LCS_IN_SteerWheelAngleSign  Interpolate=off  OutputAfterFinalValue=Setting to zero
  sourceValue_LCS_IN_axvRefMs2 : FromWorkspace  VariableName=s_LCS_IN_axvRefMs2  Interpolate=off  OutputAfterFinalValue=Setting to zero
  sourceValue_LCS_IN_ayvRefMs2 : FromWorkspace  VariableName=s_LCS_IN_ayvRefMs2  Interpolate=off  OutputAfterFinalValue=Setting to zero
  sourceValue_LCS_IN_kapTraj : FromWorkspace  VariableName=s_LCS_IN_kapTraj  Interpolate=off  OutputAfterFinalValue=Setting to zero
  sourceValue_LCS_IN_psiDtOpt : FromWorkspace  VariableName=s_LCS_IN_psiDtOpt  Interpolate=off  OutputAfterFinalValue=Setting to zero
  sourceValue_LCS_IN_vxvRefMs : FromWorkspace  VariableName=s_LCS_IN_vxvRefMs  Interpolate=off  OutputAfterFinalValue=Setting to zero
  LCS_IN_SteerWheelAng : Outport
  LCS_IN_SteerWheelAngleSign : Outport  Port=2
  LCS_IN_SteerAngOffset_deg : Outport  Port=3
  LCS_IN_vxvRefMs : Outport  Port=4
  LCS_IN_psiDtOpt : Outport  Port=5
  LCS_IN_axvRefMs2 : Outport  Port=6
  LCS_IN_ayvRefMs2 : Outport  Port=7
  LCS_IN_kapTraj : Outport  Port=8
  wires:
  sourceValue_LCS_IN_SteerWheelAng/1 -> LCS_IN_SteerWheelAng/1  "LCS_IN_SteerWheelAng"
  sourceValue_LCS_IN_SteerWheelAngleSign/1 -> LCS_IN_SteerWheelAngleSign/1  "LCS_IN_SteerWheelAngleSign"
  sourceValue_LCS_IN_SteerAngOffset_deg/1 -> LCS_IN_SteerAngOffset_deg/1  "LCS_IN_SteerAngOffset_deg"
  sourceValue_LCS_IN_vxvRefMs/1 -> LCS_IN_vxvRefMs/1  "LCS_IN_vxvRefMs"
  sourceValue_LCS_IN_psiDtOpt/1 -> LCS_IN_psiDtOpt/1  "LCS_IN_psiDtOpt"
  sourceValue_LCS_IN_axvRefMs2/1 -> LCS_IN_axvRefMs2/1  "LCS_IN_axvRefMs2"
  sourceValue_LCS_IN_ayvRefMs2/1 -> LCS_IN_ayvRefMs2/1  "LCS_IN_ayvRefMs2"
  sourceValue_LCS_IN_kapTraj/1 -> LCS_IN_kapTraj/1  "LCS_IN_kapTraj"

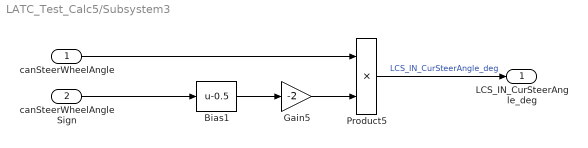
== system LATC_Test_Calc5/Subsystem3 ==
  canSteerWheelAngle : Inport
  canSteerWheelAngleSign : Inport  Port=2
  Bias1 : Bias  Bias=-0.5
  Gain5 : Gain  Gain=-2
  Product5 : Product
  LCS_IN_CurSteerAngle_deg : Outport
  wires:
  Product5/1 -> LCS_IN_CurSteerAngle_deg/1  "LCS_IN_CurSteerAngle_deg"
  canSteerWheelAngleSign/1 -> Bias1/1
  Gain5/1 -> Product5/2
  canSteerWheelAngle/1 -> Product5/1
  Bias1/1 -> Gain5/1

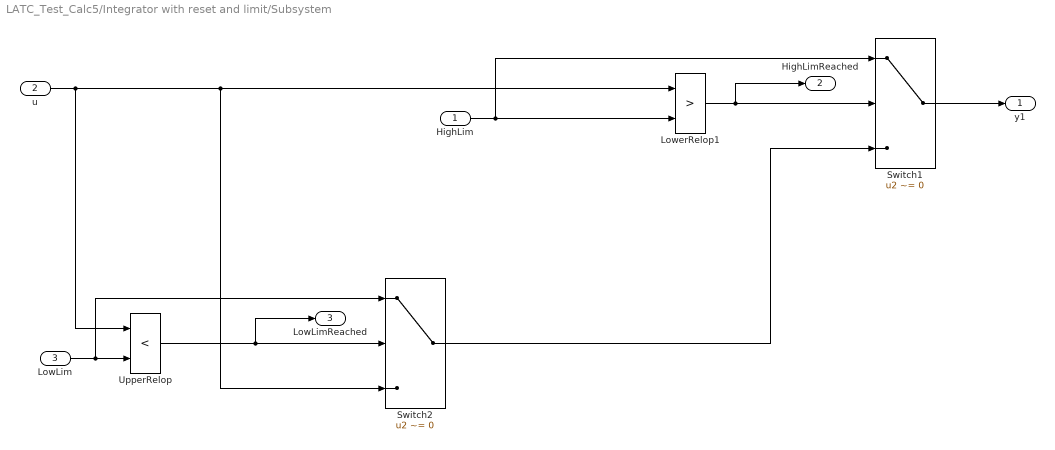
== system LATC_Test_Calc5/Integrator with reset and limit/Subsystem ==
  HighLim : Inport
  u : Inport  Port=2
  LowLim : Inport  Port=3
  LowerRelop1 : RelationalOperator  DisableCoverage=on  Operator=>  OutDataTypeStr=boolean  RndMeth=Nearest
  Switch1 : Switch  Criteria=u2 ~= 0  InputSameDT=on
      settings: AttributesFormatString=InputSameDT = %<InputSameDT>
  Switch2 : Switch  Criteria=u2 ~= 0  InputSameDT=on
      settings: AttributesFormatString=InputSameDT = %<InputSameDT>
  UpperRelop : RelationalOperator  DisableCoverage=on  Operator=<  OutDataTypeStr=boolean  RndMeth=Nearest
  y1 : Outport
  HighLimReached : Outport  Port=2
  LowLimReached : Outport  Port=3
  wires:
  Switch2/1 -> Switch1/3
  Switch1/1 -> y1/1
  HighLim/1 -> LowerRelop1/2, Switch1/1
  u/1 -> UpperRelop/1, LowerRelop1/1, Switch2/3
  LowLim/1 -> UpperRelop/2, Switch2/1
  UpperRelop/1 -> LowLimReached/1, Switch2/2
  LowerRelop1/1 -> HighLimReached/1, Switch1/2

== matlab function LATC_Test_Calc5/MATLAB Function3 ==
  data: Speed_ms input; Vy_SteerAngle_Vch output; SteerWheelAngle input; Vy_SteerAngle_Kv output; Vy_YawRate output; Critical_Spd output; CharSpd output; YawRate input; SteerChar output; Vch_Cal output
function [Vy_SteerAngle_Vch,Vy_SteerAngle_Kv,Vy_YawRate,Critical_Spd,CharSpd,SteerChar,Vch_Cal]= Vy_Calc(Speed_ms,SteerWheelAngle,YawRate)
    m = single(1720);
    L=single(2.91);
    a = single(1.27);
    b = single(1.64);
    Vch=single(23.5);
    caf = single(2*55000);
    car = single(2*75000);
    %%  根据Vy/steerAngle = K_gain，其中Kv(不足转向斜率)根据特征车速计算
    KKg1 = (Vch*Vch*Speed_ms)/((Vch^2+Vch^2)*L);
    KKg2 = (b - ((m*a*Speed_ms*Speed_ms)/(car*L)));
    K_gain = KKg1*KKg2;
    Vy_SteerAngle_Vch = (SteerWheelAngle/15.5/57.3)*K_gain;
    %%  根据Vy/steerAngle = KK_gain，其中Kv(不足转向斜率)根据前后轮胎刚度计算
    Kg1 = (car*caf*b*L*Speed_ms)-(caf*a*m*Speed_ms*Speed_ms*Speed_ms);
    Kg2 = (car*caf*L*L)+(m*Speed_ms*Speed_ms*(b*car-a*caf));
    KK_gain = Kg1/Kg2;
    Vy_SteerAngle_Kv = KK_gain*(SteerWheelAngle/15.5/57.3);
    %%  根据Vy/YawRate = KKK_gain
    KKK_gain = (b-(m*a*Speed_ms*Speed_ms)/(car*L));
    Vy_YawRate = (YawRate)*KKK_gain;
    %%  根据Vy/YawRate = KKK_gain,质心侧偏角为0时的，质心侧偏角的临界车速值，超过该车速质心侧偏角会反向，Vy也会反向
    Critical_Spd = sqrt((car*L*b)/(m*a));
    %%  由于前后轮胎刚度不确定，通常可时实际测得CharSpd，通过调整前后轮胎刚度使计算得到的车辆特征车速尽可能接近测试值，进而使设定的轮胎刚度更加接近真实值
    CharSpd= sqrt(1/((m/(L*L))*((b/caf)-(a/car)))); % 车辆特征车速（过渡转向和转向不足的临界车速，ESP提供）
    %% 转向性质表征 小于零为转向不足，大于零为转向过度
    SteerChar = sign(a*caf-b*car);
    %% 理论计算特征车速
    SM = abs(-((a*caf-b*car)/(L*(caf+car))));%静态裕度
    temp = (2*L*(caf/2)*(car/2))/(m*((caf/2)+(car/2)));
    Vch_Cal = sqrt(temp*(1/SM));
    %%
    Veh_Speed = 10;
    veh_params.wheel_base = single(2.92);               %轴距, m
    veh_params.Vch = single(23.5);                      %特征车速
    veh_params.mu = single(0.85);                       %路面摩擦限制
    veh_params.max_acceleration = single(2);            %车辆最大加速度
    veh_params.max_deceleration = single(-2);           %车辆最大减速度
    veh_params.left_steer_ratio = 1;     %车辆左侧转向传动比%
    veh_params.right_steer_ratio = 1;   %车辆右侧转向传动比%
    veh_params.cf = single(55000);                      %车辆前轮侧偏刚度N/rad(两侧轮胎等效为一个*2)
    veh_params.cr = single(75000);                      %车辆后轮侧偏刚度N/rad
    veh_params.clf = single(5000);                      %车辆前轮纵向刚度(两侧轮胎等效为一个*2)
    veh_params.clr = single(5000);                      %车辆后轮纵向刚度
    
    veh_params.mass_fl = single(520);                   %车辆左前轮负重
    veh_params.mass_fr = single(520);                   %车辆右前轮负重
    veh_params.mass_rl = single(520);                   %车辆左后轮负重
    veh_params.mass_rr = single(520);                   %车辆右后轮负重
    veh_params.Sf = single(0.2);                        %车辆前轮滑移率
    veh_params.Sr = single(0.2);                        %车辆后轮滑移率
   %% 2.控制参数计算
    mass_front =  veh_params.mass_fl + veh_params.mass_fr;
    mass_rear  =  veh_params.mass_rl + veh_params.mass_rr;
    mass =  mass_front + mass_rear;
    lf = veh_params.wheel_base * (single(1.0) - mass_front / mass);% distance from front tires to cg, m 前轴到质心的距离
    lr = veh_params.wheel_base * (single(1.0) - mass_rear / mass);% distance from rear tires to cg, m  后轴到质心的距离
    iz = lf * lf * mass_front + lr * lr * mass_rear; % 转动惯量
    %---------------------------求车辆响应增益---------------------------%
    % % 车辆模型，状态为[v,wr]
    % 求车辆响应增益
    Veh_Speed = 10;
    AAr = [(2*veh_params.cf+2*veh_params.cr)/Veh_Speed,((2*veh_params.cf*lf-2*veh_params.cr*lr)/Veh_Speed)+mass*Veh_Speed;
           (2*veh_params.cf*lf-2*veh_params.cr*lr)/Veh_Speed,(2*veh_params.cf*lf^2+2*veh_params.cr*lr^2)/Veh_Speed];
    BBr = [2*veh_params.cf;2*veh_params.cf*lf];
    a11 = AAr(1,1);
    a12 = AAr(1,2);
    a21 = AAr(2,1);
    a22 = AAr(2,2);
    b1 = BBr(1);
    b2 = BBr(2);
    %Ta = a11+a22;
    Da = a11*a22-a12*a21;
    
    Gr = (b2*a11-b1*a21)/Da; % 稳态横摆角速度增益，理想化增益是偏大，因为轮胎侧偏刚度会变小(此处的稳态横摆角速度增益是δ/wr，书中的公式为wr/δ范围0.16~0.33)
    % Gb = (b1.*a22-b2.*a12)./Da; % 稳态质心侧偏角增益，理想化增益是偏大，因为轮胎侧偏刚度会变小
    % Gay = Gr*Veh_Speed; % 稳态侧向加速度增益，理想化增益是偏大，因为轮胎侧偏刚度会变小，此处公式错误应该如下
    Gv = (b1*a22-b2*a12)/Da;% 稳态横向速度增益，理想化增益是偏大，因为轮胎侧偏刚度会变小
    Gay = Veh_Speed/Gr; % 稳态侧向加速度增益，理想化增益是偏大，因为轮胎侧偏刚度会变小。
    Gay2 = Veh_Speed*Gr;

    A = 5/57.3;
    AA = A* Gay2;
    AAA = A*Gr;

    AAAA = A*Gv;
    B=10;

    CC = 10
end
